simulink model "Interp"  (Simulink 7.1)
settings: Solver=ode45  SolverMode=SingleTasking  StartTime=0.0  StopTime=60.0  MaxStep=.05  RelTol=1e-3  AbsTol=1e-6
undefined symbols (not defined in the file): a, b, c, d
settings Model: Creator=vise  LastModifiedBy=vise  ExtModeTrigMode=oneshot  ExtModeArmWhenConnect=off  ExtModeAutoUpdateStatusClock=off
settings DataIOCC: LimitDataPoints=off
settings OptimizationCC: BooleanDataType=off
settings DebuggingCC: SaveWithParameterizedLinksMsg=none  SignalResolutionControl=TryResolveAllWithWarning  SolverPrmCheckMsg=none  MultiTaskDSMMsg=warning  MultiTaskCondExecSysMsg=none  StrictBusMsg=None
settings HardwareCC: TargetUnknown=on
settings RTWCC: TemplateMakefile=grt_unix.tmf  IncludeERTFirstTime=on

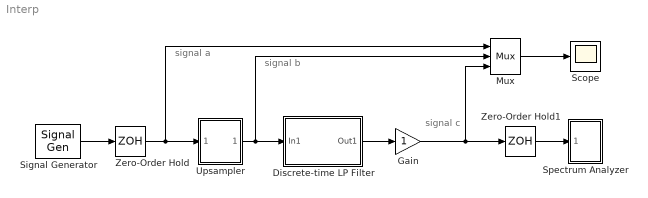
== system Interp ==
  note: signal c
  note: signal b
  note: signal a
  Discrete-time LP Filter : Subsystem  mask(butter){@1=3.14159, @2=10, @3=1}
      mask prompts: @1 "Cutoff frequency (0 to pi):"; @2 "Order:"; @3 "Sample time:"
      mask help:
      | Butterworth low pass filter.
      | (Requires Signal Processing Toolbox)
      mask init:
      | [a,b,c,d]=butter(@2,@1/pi); ts=@3; [num,den]=ss2tf(a,b,c,d,1); if (@2 <= 8), [a,b,c,d]=tf2ss(num,den); end; h=freqz(num,den,64);
      mask Help: IIR Butterworth low pass filter using MATLAB's butter command.
      mask Display: plot(1:64,abs(h))
  Gain : Gain  SaturateOnIntegerOverflow=on  OutDataTypeStr=Inherit: Same as input  ParamDataTypeStr=Inherit: Same as input
  Mux : Mux  Inputs=3
  Scope : Scope
      settings: TickLabels=on  TimeRange=30  YMin=-1.5  YMax=1.5  DataFormat=Array
  Signal Generator : SignalGenerator  Amplitude=1.000000  Frequency=0.1
  Spectrum Analyzer : Subsystem  mask(Spectrum analyzer.){@1=1024, @2=.05, @3=10}
      mask prompts: @1 "Number of sample points:"; @2 "Sampling period (sec):"; @3 "Plotting Period (sec):"
      mask init:
      | N=@1; T_s=@2;plot_period=@3;
      mask Help: EE438 Lab utility; See Prof. Bouman.
      mask Display: plot(0,0,100,100,[14,91,91,14,14],[86,86,40,40,86],[85,82,80,79,75,67,63,60,57,53,41,36,33,27,24],[49,50,53,50,49,51,54,66,54,50,50,52,81,51,49])
  Upsampler : Subsystem  mask(D-T interpolator){@1=1, @2=1}
      mask prompts: @1 "Input sampling period:"; @2 "Upsampling factor:"
      mask init:
      | T=@1;L=@2;
      mask Display: disp('L')
  Zero-Order Hold : ZeroOrderHold
  Zero-Order Hold1 : ZeroOrderHold  SampleTime=.05
  wires:
  Zero-Order Hold1/1 -> Spectrum Analyzer/1(input signal)
  Mux/1 -> Scope/1
  Gain/1 -> Zero-Order Hold1/1, Mux/3
  Discrete-time LP Filter/1(Out1) -> Gain/1
  Zero-Order Hold/1 -> Mux/1, Upsampler/1(in_1)
  Upsampler/1(out_1) -> Discrete-time LP Filter/1(In1), Mux/2
  Signal Generator/1 -> Zero-Order Hold/1

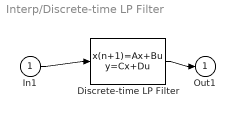
== system Interp/Discrete-time LP Filter ==
  In1 : Inport
  Discrete-time LP Filter : DiscreteStateSpace  A=a  B=b  C=c  D=d  SampleTime=ts
  Out1 : Outport
  wires:
  In1/1 -> Discrete-time LP Filter/1
  Discrete-time LP Filter/1 -> Out1/1

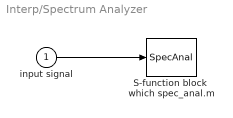
== system Interp/Spectrum Analyzer ==
  input signal : Inport
  S-function block  which spec_anal.m : S-Function  FunctionName=SpecAnal  Parameters=N,T_s,plot_period  EnableBusSupport=off
  wires:
  input signal/1 -> S-function block  which spec_anal.m/1

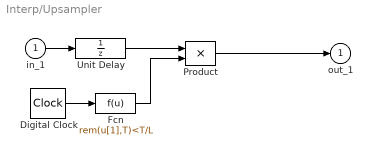
== system Interp/Upsampler ==
  in_1 : Inport
  Digital Clock : DigitalClock  SampleTime=T/L
  Fcn : Fcn  Expr=rem(u[1],T)<T/L
  Product : Product  SaturateOnIntegerOverflow=on  RndMeth=Zero  InputSameDT=on  OutDataTypeStr=Inherit: Same as first input
  Unit Delay : UnitDelay  SampleTime=T/L
  out_1 : Outport  InitialOutput=0
  wires:
  Product/1 -> out_1/1
  Fcn/1 -> Product/2
  Unit Delay/1 -> Product/1
  in_1/1 -> Unit Delay/1
  Digital Clock/1 -> Fcn/1
